simulink model "simTurboLibMat1_2"  (R2016b)
settings: Solver=VariableStepAuto  StartTime=0.0  StopTime=10  RelTol=1e-3
values from neighbouring files (symbols this model uses):
  variance = 1/(2*r*10^(vectEbNo(i)/10))    [TC_CCSDS_1_2.m]    (also in TC_CCSDS_1_3.m; TC_CCSDS_1_4.m; TC_CCSDS_1_6.m)
undefined symbols (not defined in the file or in its folder): blockLen
libraries: commsequence2 x4, commchan3 x2, commrandsrc3 x2, commcnvcod2 x2, commutil2 x2, commsink2 x1, dspsigops x1
settings Model: Creator=migm2  LastModifiedBy=migm2

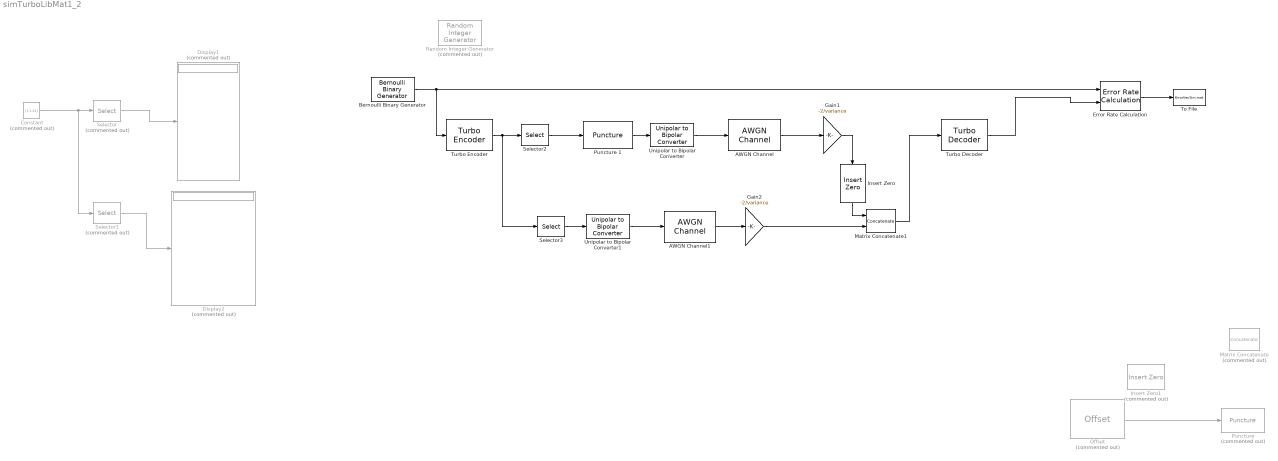
== system simTurboLibMat1_2 ==
  AWGN Channel : commchan3/AWGN Channel  InputProcessing=Columns as channels (frame based)  seed=67  noiseMode=Variance from mask  EbNodB=EbNo  EsNodB=10  SNRdB=10  bitsPerSym=1  Ps=1  Tsym=1/blockLen  variance=variance
  AWGN Channel1 : commchan3/AWGN Channel  InputProcessing=Columns as channels (frame based)  seed=67  noiseMode=Variance from mask  EbNodB=EbNo  EsNodB=10  SNRdB=10  bitsPerSym=1  Ps=1  Tsym=1/blockLen  variance=variance
  Bernoulli Binary Generator : commrandsrc3/Bernoulli Binary Generator  ProbabilityOfZero=0.5  SeedSource=Parameter  Seed=12345  SampleTime=1/blockLen  SamplesPerFrame=blockLen  OutputDataType=double  SimulateUsing=Interpreted execution
  Constant : Constant  Commented=on  Value=[1:1:31]
  Display1 : Display  Commented=on
  Display2 : Display  Commented=on
  Error Rate Calculation : commsink2/Error Rate Calculation  N=0  st_delay=0  cp_mode=Entire frame  subframe=[]  PMode=Port  WsName=ErrorVecSim  RsMode2=off  stop=off  numErr=100  maxBits=1e6
  Gain1 : Gain  Gain=-2/variance  SaturateOnIntegerOverflow=on  OutDataTypeStr=Inherit: Same as input  ParamDataTypeStr=Inherit: Same as input
  Gain2 : Gain  Gain=-2/variance  SaturateOnIntegerOverflow=on  OutDataTypeStr=Inherit: Same as input  ParamDataTypeStr=Inherit: Same as input
  Insert Zero : commsequence2/Insert Zero  insertZeroVector=punct
  Insert Zero1 : commsequence2/Insert Zero  Commented=on  insertZeroVector=[1 1 0 1 0 1].'
  Matrix Concatenate : Concatenate  Commented=on  Mode=Multidimensional array  ConcatenateDimension=2
  Matrix Concatenate1 : Concatenate  ConcatenateDimension=2
  Offset : dspsigops/Offset  Commented=on  mode=Keep beginning samples  numDatOffPair=1  outWidthSpec=User-defined  outWidth=5352  actionOutRange=Clip
  "Puncture " : commsequence2/Puncture  Commented=on  punctureVector=[1 1 0 1 0 1].'
  Puncture 1 : commsequence2/Puncture  punctureVector=punct
  Random Integer Generator : commrandsrc3/Random Integer Generator  Commented=on  SetSize=1  SeedSource=Parameter  Seed=12345  SampleTime=1/blockLen  SamplesPerFrame=blockLen  OutputDataType=double  SimulateUsing=Interpreted execution
  Selector : Selector  Commented=on  InputPortWidth=31  IndexOptions=Starting index (dialog)  Indices=1  OutputSizes=15
  Selector1 : Selector  Commented=on  InputPortWidth=31  IndexOptions=Starting index (dialog)  Indices=16  OutputSizes=16
  Selector2 : Selector  InputPortWidth=blockLen*3+16  IndexOptions=Starting index (dialog)  Indices=1  OutputSizes=blockLen*3
  Selector3 : Selector  InputPortWidth=blockLen*3+16  IndexOptions=Starting index (dialog)  Indices=blockLen*3+1  OutputSizes=16
  To File : ToFile  Filename=ErrorVecSim.mat  MatrixName=ErrorVecSim
  Turbo Decoder : commcnvcod2/Turbo Decoder  TrellisStructure=trellis  InterleaverIndicesSource=Property  InterleaverIndices=indInter  Algorithm=True APP  NumScalingBits=3  NumIterations=numIter  SimulateUsing=Interpreted execution
  Turbo Encoder : commcnvcod2/Turbo Encoder  TrellisStructure=trellis  InterleaverIndicesSource=Property  InterleaverIndices=indInter  SimulateUsing=Interpreted execution
  Unipolar to Bipolar Converter : commutil2/Unipolar to Bipolar Converter  M=2  polarity=Negative  dataType=double
  Unipolar to Bipolar Converter1 : commutil2/Unipolar to Bipolar Converter  M=2  polarity=Negative  dataType=double
  wires:
  Turbo Decoder/1 -> Error Rate Calculation/2
  Bernoulli Binary Generator/1 -> Turbo Encoder/1, Error Rate Calculation/1
  AWGN Channel/1 -> Gain1/1
  Unipolar to Bipolar Converter/1 -> AWGN Channel/1
  Turbo Encoder/1 -> Selector3/1, Selector2/1
  Offset/1 -> "Puncture "/1
  Constant/1 -> Selector1/1, Selector/1
  Selector/1 -> Display1/1
  Selector1/1 -> Display2/1
  Selector2/1 -> Puncture 1/1
  AWGN Channel1/1 -> Gain2/1
  Unipolar to Bipolar Converter1/1 -> AWGN Channel1/1
  Gain2/1 -> Matrix Concatenate1/2
  Selector3/1 -> Unipolar to Bipolar Converter1/1
  Gain1/1 -> Insert Zero/1
  Matrix Concatenate1/1 -> Turbo Decoder/1
  Insert Zero/1 -> Matrix Concatenate1/1
  Puncture 1/1 -> Unipolar to Bipolar Converter/1
  Error Rate Calculation/1 -> To File/1
